simulink model "buck_boost_DCDC_sim"  (R2020a)
settings: Solver=FixedStepAuto  StartTime=0.0  StopTime=sim_duration  FixedStep=time_step  RelTol=1e-3
undefined symbols (not defined in the file): beta, C, E, K_fl, K_smc_0, L, noise_enable, phi, prefiltar_enable, R, R_dot_enable, sigma_noise, step_poremecaj, step_ref, t_poremecaj, t_ref, time_step, w_diff, w_prefiltar, x_2e
settings Model: Creator=HP  LastModifiedBy=HP

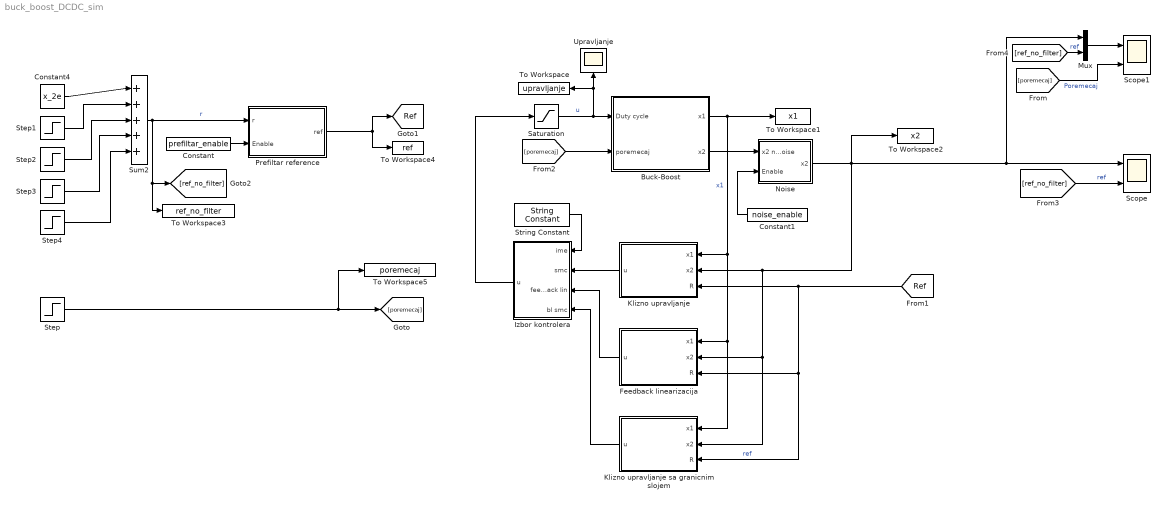
== system buck_boost_DCDC_sim ==
  Buck-Boost : Subsystem
  Constant : Constant  Value=prefiltar_enable
  Constant1 : Constant  Value=noise_enable
  Constant4 : Constant  Value=x_2e
  Feedback linearizacija : Subsystem
  Izbor kontrolera : Subsystem
  Klizno upravljanje : Subsystem
  Klizno upravljanje sa granicnim slojem : Subsystem
  Mux : Mux  Inputs=2
  Noise : Subsystem
  Prefiltar reference : Subsystem
  Saturation : Saturate  UpperLimit=1  LowerLimit=0
  Scope : Scope  NumInputPorts=2
  Scope1 : Scope  NumInputPorts=2
  Step : Step  Time=t_poremecaj(1)  After=step_poremecaj(1)  SampleTime=0
  Step1 : Step  Time=t_ref(1)  After=step_ref(1)  SampleTime=0
  Step2 : Step  Time=t_ref(2)  After=step_ref(2)  SampleTime=0
  Step3 : Step  Time=t_ref(3)  After=step_ref(3)  SampleTime=0
  Step4 : Step  Time=t_ref(4)  After=step_ref(4)  SampleTime=0
  String Constant : StringConstant  String=ime_kontrolera
  Sum2 : Sum  Inputs=|+++++
  To Workspace : ToWorkspace  VariableName=upravljanje  SaveFormat=Timeseries  SampleTime=-1
  To Workspace1 : ToWorkspace  VariableName=x1  SaveFormat=Timeseries  SampleTime=-1
  To Workspace2 : ToWorkspace  VariableName=x2  SaveFormat=Timeseries  SampleTime=-1
  To Workspace3 : ToWorkspace  VariableName=ref_no_filter  SaveFormat=Timeseries  SampleTime=-1
  To Workspace4 : ToWorkspace  VariableName=ref  SaveFormat=Timeseries  SampleTime=-1
  To Workspace5 : ToWorkspace  VariableName=poremecaj  SaveFormat=Timeseries  SampleTime=-1
  Upravljanje : Scope
  tag scope: Ref=global
  wires:
  [ref_no_filter] -> Scope/2  "ref"
  Step1/1 -> Sum2/2
  Constant4/1 -> Sum2/1
  Saturation/1 -> Buck-Boost/1(Duty cycle), To Workspace/1, Upravljanje/1  "u"
  Step2/1 -> Sum2/3
  Buck-Boost/1(x1) -> Klizno upravljanje sa granicnim slojem/1(x1), Feedback linearizacija/1(x1), Klizno upravljanje/1(x1), To Workspace1/1  "x1"
  [Ref] -> Klizno upravljanje sa granicnim slojem/3(R), Feedback linearizacija/3(R), Klizno upravljanje/3(R)  "ref"
  Step/1 -> To Workspace5/1, [poremecaj]
  [poremecaj] -> Buck-Boost/2(poremecaj)
  Sum2/1 -> Prefiltar reference/1(r), [ref_no_filter], To Workspace3/1  "r"
  String Constant/1 -> Izbor kontrolera/1(ime)
  Izbor kontrolera/1(u) -> Saturation/1
  Klizno upravljanje/1(u) -> Izbor kontrolera/2(smc)
  Feedback linearizacija/1(u) -> Izbor kontrolera/3(feedback lin)
  Klizno upravljanje sa granicnim slojem/1(u) -> Izbor kontrolera/4(bl smc)
  Step3/1 -> Sum2/4
  Step4/1 -> Sum2/5
  Mux/1 -> Scope1/1
  [ref_no_filter] -> Mux/2  "ref"
  [poremecaj] -> Scope1/2  "Poremecaj"
  Noise/1(x2) -> Mux/1, Scope/1, To Workspace2/1, Klizno upravljanje sa granicnim slojem/2(x2), Feedback linearizacija/2(x2), Klizno upravljanje/2(x2)
  Buck-Boost/2(x2) -> Noise/1(x2 no noise)
  Constant1/1 -> Noise/2(Enable)
  Prefiltar reference/1(ref) -> [Ref], To Workspace4/1
  Constant/1 -> Prefiltar reference/2(Enable)

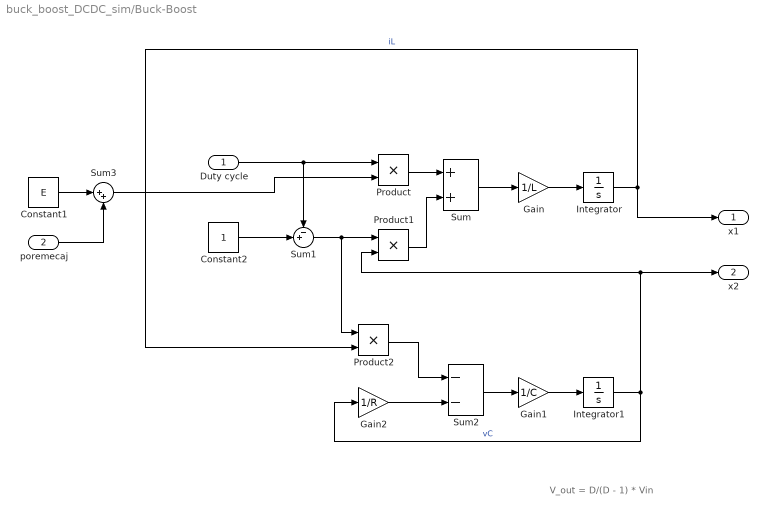
== system buck_boost_DCDC_sim/Buck-Boost ==
  note: V_out = D/(D - 1) * Vin
  Duty cycle : Inport
  poremecaj : Inport  Port=2
  Constant1 : Constant  Value=E
  Constant2 : Constant
  Gain : Gain  Gain=1/L
  Gain1 : Gain  Gain=1/C
  Gain2 : Gain  Gain=1/R
  Integrator : Integrator  InitialCondition=1e-3
  Integrator1 : Integrator  InitialCondition=-1e-3
  Product : Product
  Product1 : Product
  Product2 : Product
  Sum : Sum
  Sum1 : Sum  Inputs=-+|
  Sum2 : Sum  Inputs=--
  Sum3 : Sum  Inputs=|++
  x1 : Outport
  x2 : Outport  Port=2
  wires:
  Product/1 -> Sum/1
  Product1/1 -> Sum/2
  Sum2/1 -> Gain1/1
  Integrator1/1 -> Gain2/1, x2/1, Product1/2  "vC"
  Gain1/1 -> Integrator1/1
  Constant2/1 -> Sum1/2
  Integrator/1 -> x1/1, Product2/2  "iL"
  Sum/1 -> Gain/1
  Gain2/1 -> Sum2/2
  Sum1/1 -> Product2/1, Product1/1
  Duty cycle/1 -> Sum1/1, Product/1
  Product2/1 -> Sum2/1
  Gain/1 -> Integrator/1
  Constant1/1 -> Sum3/1
  Sum3/1 -> Product/2
  poremecaj/1 -> Sum3/2

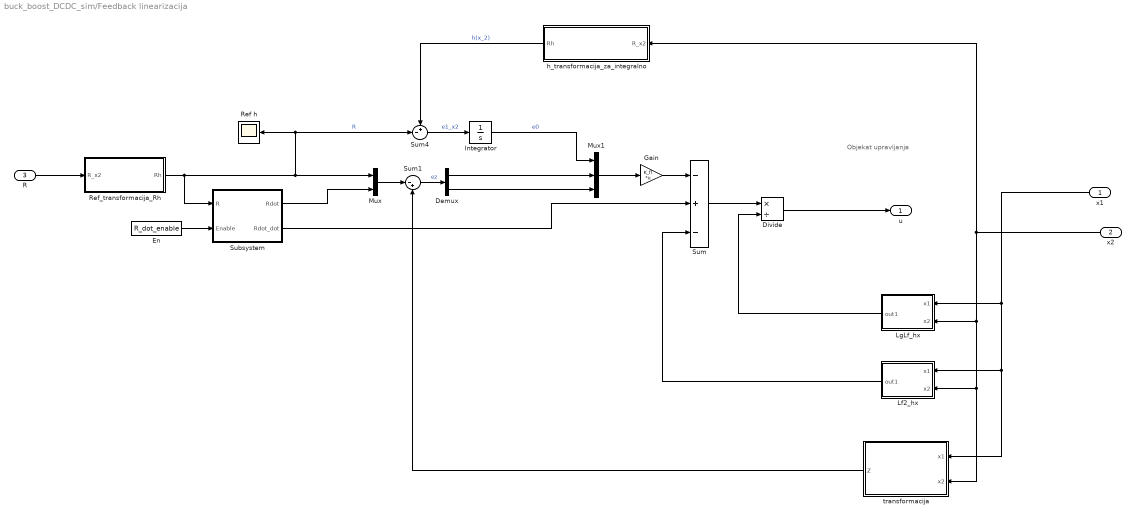
== system buck_boost_DCDC_sim/Feedback linearizacija ==
  note: Objekat upravljanja
  x1 : Inport
  x2 : Inport  Port=2
  R : Inport  Port=3
  Demux : Demux  Outputs=2
  Divide : Product  Inputs=*/
  En : Constant  Value=R_dot_enable
  Gain : Gain  Gain=K_fl  Multiplication=Matrix(K*u)
  Integrator : Integrator
  Lf2_hx : MATLAB Function  TreatAsAtomicUnit=on
  LgLf_hx : MATLAB Function  TreatAsAtomicUnit=on
  Mux : Mux  Inputs=2
  Mux1 : Mux  Inputs=3
  Ref h : Scope
  Ref_transformacija_Rh : MATLAB Function  TreatAsAtomicUnit=on
  Subsystem : Subsystem
  Sum : Sum  Inputs=-+-
  Sum1 : Sum  Inputs=|-+
  Sum4 : Sum  Inputs=+-|
  h_transformacija_za_integralno : MATLAB Function  TreatAsAtomicUnit=on
  transformacija : MATLAB Function  TreatAsAtomicUnit=on
  u : Outport
  wires:
  Subsystem/1(Rdot) -> Mux/2
  Divide/1 -> u/1
  Ref_transformacija_Rh/1(Rh) -> Sum4/2, Ref h/1, Mux/1, Subsystem/1(R)  "R"
  x1/1 -> LgLf_hx/1(x1), Lf2_hx/1(x1), transformacija/1(x1)
  Mux/1 -> Sum1/1
  LgLf_hx/1(out1) -> Divide/2
  x2/1 -> h_transformacija_za_integralno/1(R_x2), LgLf_hx/2(x2), Lf2_hx/2(x2), transformacija/2(x2)
  Demux/1 -> Mux1/2
  Sum1/1 -> Demux/1  "ez"
  Gain/1 -> Sum/1
  Subsystem/2(Rdot_dot) -> Sum/2
  Lf2_hx/1(out1) -> Sum/3
  En/1 -> Subsystem/2(Enable)
  transformacija/1(Z) -> Sum1/2
  R/1 -> Ref_transformacija_Rh/1(R_x2)
  Sum/1 -> Divide/1
  Mux1/1 -> Gain/1
  Integrator/1 -> Mux1/1  "e0"
  Sum4/1 -> Integrator/1  "e1_x2"
  Demux/2 -> Mux1/3
  h_transformacija_za_integralno/1(Rh) -> Sum4/1  "h(x_2)"

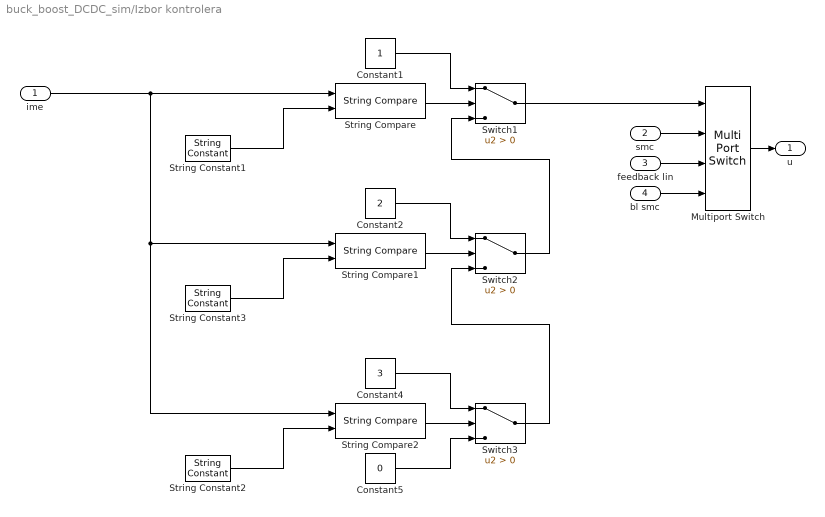
== system buck_boost_DCDC_sim/Izbor kontrolera ==
  ime : Inport
  smc : Inport  Port=2
  feedback lin : Inport  Port=3
  bl smc : Inport  Port=4
  Constant1 : Constant
  Constant2 : Constant  Value=2
  Constant4 : Constant  Value=3
  Constant5 : Constant  Value=0
  Multiport Switch : MultiPortSwitch
  String Compare : StringCompare
  String Compare1 : StringCompare
  String Compare2 : StringCompare
  String Constant1 : StringConstant  String="\"smc\""
  String Constant2 : StringConstant  String="\"bl smc\""
  String Constant3 : StringConstant  String="\"fbl\""
  Switch1 : Switch  Criteria=u2 > Threshold
  Switch2 : Switch  Criteria=u2 > Threshold
  Switch3 : Switch  Criteria=u2 > Threshold
  u : Outport
  wires:
  String Compare1/1 -> Switch2/2
  Switch1/1 -> Multiport Switch/1
  String Constant1/1 -> String Compare/2
  String Constant3/1 -> String Compare1/2
  Constant1/1 -> Switch1/1
  Constant2/1 -> Switch2/1
  Switch2/1 -> Switch1/3
  String Compare/1 -> Switch1/2
  feedback lin/1 -> Multiport Switch/3
  Multiport Switch/1 -> u/1
  smc/1 -> Multiport Switch/2
  bl smc/1 -> Multiport Switch/4
  Constant5/1 -> Switch3/3
  ime/1 -> String Compare/1, String Compare2/1, String Compare1/1
  String Compare2/1 -> Switch3/2
  String Constant2/1 -> String Compare2/2
  Constant4/1 -> Switch3/1
  Switch3/1 -> Switch2/3

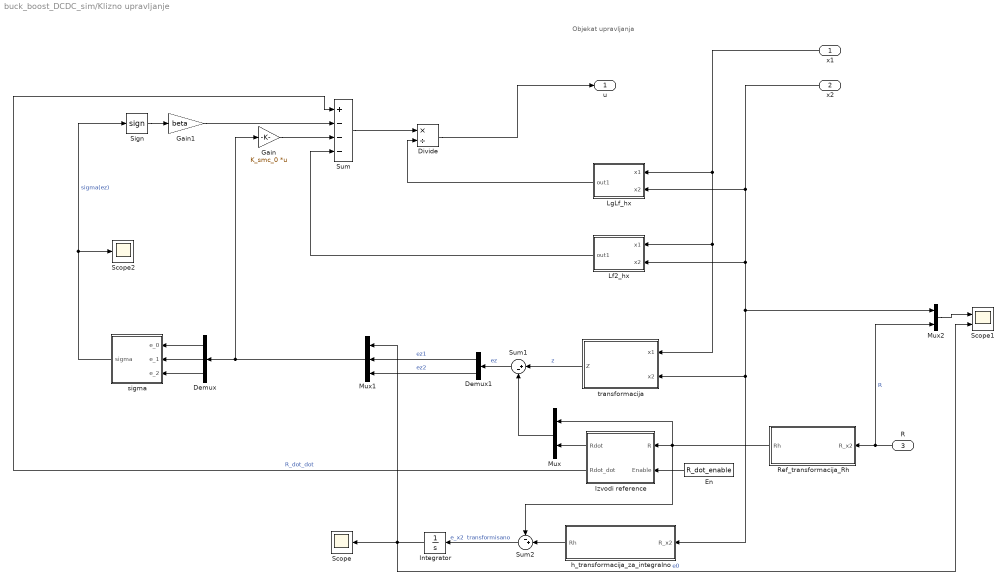
== system buck_boost_DCDC_sim/Klizno upravljanje ==
  note: Objekat upravljanja
  x1 : Inport
  x2 : Inport  Port=2
  R : Inport  Port=3
  Demux : Demux  Outputs=3
  Demux1 : Demux  Outputs=2
  Divide : Product  Inputs=*/
  En : Constant  Value=R_dot_enable
  Gain : Gain  Gain=K_smc_0  Multiplication=Matrix(K*u)
  Gain1 : Gain  Gain=beta
  Integrator : Integrator
  Izvodi reference : Subsystem
  Lf2_hx : MATLAB Function  TreatAsAtomicUnit=on
  LgLf_hx : MATLAB Function  TreatAsAtomicUnit=on
  Mux : Mux  Inputs=2
  Mux1 : Mux  Inputs=3
  Mux2 : Mux  Inputs=2
  Ref_transformacija_Rh : MATLAB Function  TreatAsAtomicUnit=on
  Scope : Scope
  Scope1 : Scope  NumInputPorts=2
  Scope2 : Scope
  Sign : Signum
  Sum : Sum  Inputs=+---
  Sum1 : Sum  Inputs=|+-
  Sum2 : Sum  Inputs=-+|
  h_transformacija_za_integralno : MATLAB Function  TreatAsAtomicUnit=on
  sigma : MATLAB Function  TreatAsAtomicUnit=on
  transformacija : MATLAB Function  TreatAsAtomicUnit=on
  u : Outport
  wires:
  x1/1 -> LgLf_hx/1(x1), transformacija/1(x1), Lf2_hx/1(x1)
  x2/1 -> Mux2/1, h_transformacija_za_integralno/1(R_x2), transformacija/2(x2), Lf2_hx/2(x2), LgLf_hx/2(x2)
  Divide/1 -> u/1
  LgLf_hx/1(out1) -> Divide/2
  Sum/1 -> Divide/1
  Lf2_hx/1(out1) -> Sum/4
  Gain/1 -> Sum/3
  transformacija/1(Z) -> Sum1/1  "z"
  sigma/1(sigma) -> Sign/1, Scope2/1  "sigma(ez)"
  Sign/1 -> Gain1/1
  Gain1/1 -> Sum/2
  En/1 -> Izvodi reference/2(Enable)
  R/1 -> Mux2/2, Ref_transformacija_Rh/1(R_x2)  "R"
  Izvodi reference/1(Rdot) -> Mux/2
  Mux/1 -> Sum1/2
  Izvodi reference/2(Rdot_dot) -> Sum/1  "R_dot_dot"
  Ref_transformacija_Rh/1(Rh) -> Sum2/1, Mux/1, Izvodi reference/1(R)
  Mux1/1 -> Gain/1, Demux/1
  Sum1/1 -> Demux1/1  "ez"
  Demux1/1 -> Mux1/2  "ez1"
  Demux1/2 -> Mux1/3  "ez2"
  h_transformacija_za_integralno/1(Rh) -> Sum2/2
  Sum2/1 -> Integrator/1  "e_x2  transformisano"
  Demux/1 -> sigma/1(e_0)
  Demux/2 -> sigma/2(e_1)
  Demux/3 -> sigma/3(e_2)
  Integrator/1 -> Scope1/2, Scope/1, Mux1/1  "e0"
  Mux2/1 -> Scope1/1

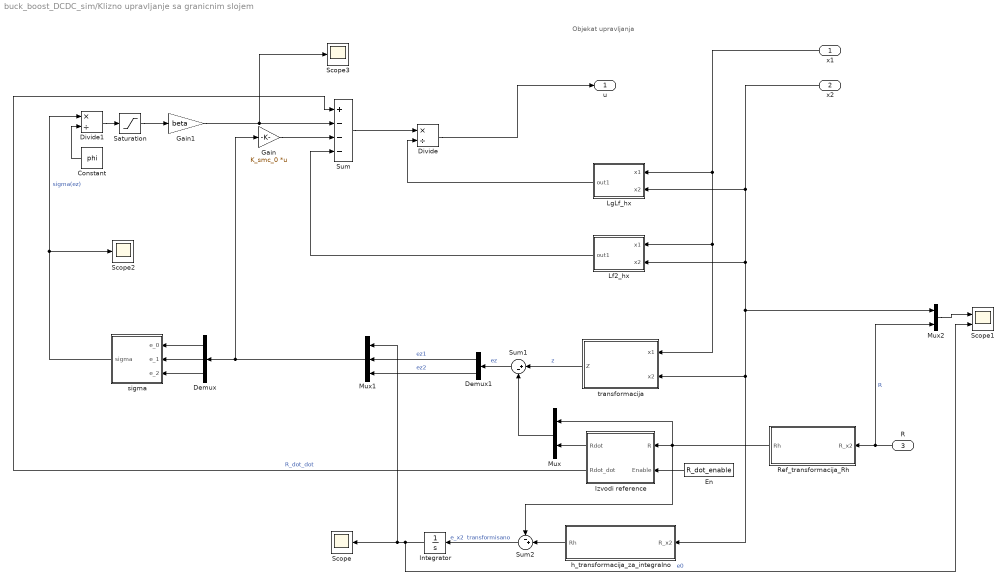
== system buck_boost_DCDC_sim/Klizno upravljanje sa granicnim slojem ==
  note: Objekat upravljanja
  x1 : Inport
  x2 : Inport  Port=2
  R : Inport  Port=3
  Constant : Constant  Value=phi
  Demux : Demux  Outputs=3
  Demux1 : Demux  Outputs=2
  Divide : Product  Inputs=*/
  Divide1 : Product  Inputs=*/
  En : Constant  Value=R_dot_enable
  Gain : Gain  Gain=K_smc_0  Multiplication=Matrix(K*u)
  Gain1 : Gain  Gain=beta
  Integrator : Integrator
  Izvodi reference : Subsystem
  Lf2_hx : MATLAB Function  TreatAsAtomicUnit=on
  LgLf_hx : MATLAB Function  TreatAsAtomicUnit=on
  Mux : Mux  Inputs=2
  Mux1 : Mux  Inputs=3
  Mux2 : Mux  Inputs=2
  Ref_transformacija_Rh : MATLAB Function  TreatAsAtomicUnit=on
  Saturation : Saturate  UpperLimit=1  LowerLimit=-1
  Scope : Scope
  Scope1 : Scope  NumInputPorts=2
  Scope2 : Scope
  Scope3 : Scope
  Sum : Sum  Inputs=+---
  Sum1 : Sum  Inputs=|+-
  Sum2 : Sum  Inputs=-+|
  h_transformacija_za_integralno : MATLAB Function  TreatAsAtomicUnit=on
  sigma : MATLAB Function  TreatAsAtomicUnit=on
  transformacija : MATLAB Function  TreatAsAtomicUnit=on
  u : Outport
  wires:
  x1/1 -> LgLf_hx/1(x1), transformacija/1(x1), Lf2_hx/1(x1)
  x2/1 -> Mux2/1, h_transformacija_za_integralno/1(R_x2), transformacija/2(x2), Lf2_hx/2(x2), LgLf_hx/2(x2)
  Divide/1 -> u/1
  LgLf_hx/1(out1) -> Divide/2
  Sum/1 -> Divide/1
  Lf2_hx/1(out1) -> Sum/4
  Gain/1 -> Sum/3
  transformacija/1(Z) -> Sum1/1  "z"
  sigma/1(sigma) -> Divide1/1, Scope2/1  "sigma(ez)"
  Saturation/1 -> Gain1/1
  Gain1/1 -> Scope3/1, Sum/2
  En/1 -> Izvodi reference/2(Enable)
  R/1 -> Mux2/2, Ref_transformacija_Rh/1(R_x2)  "R"
  Izvodi reference/1(Rdot) -> Mux/2
  Mux/1 -> Sum1/2
  Izvodi reference/2(Rdot_dot) -> Sum/1  "R_dot_dot"
  Ref_transformacija_Rh/1(Rh) -> Sum2/1, Mux/1, Izvodi reference/1(R)
  Mux1/1 -> Gain/1, Demux/1
  Sum1/1 -> Demux1/1  "ez"
  Demux1/1 -> Mux1/2  "ez1"
  Demux1/2 -> Mux1/3  "ez2"
  h_transformacija_za_integralno/1(Rh) -> Sum2/2
  Sum2/1 -> Integrator/1  "e_x2  transformisano"
  Demux/1 -> sigma/1(e_0)
  Demux/2 -> sigma/2(e_1)
  Demux/3 -> sigma/3(e_2)
  Integrator/1 -> Scope1/2, Scope/1, Mux1/1  "e0"
  Mux2/1 -> Scope1/1
  Divide1/1 -> Saturation/1
  Constant/1 -> Divide1/2

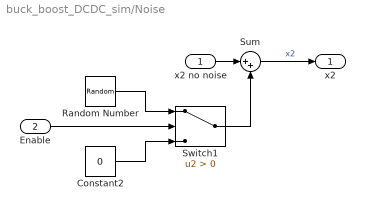
== system buck_boost_DCDC_sim/Noise ==
  x2 no noise : Inport
  Enable : Inport  Port=2
  Constant2 : Constant  Value=0
  Random Number : RandomNumber  Variance=sigma_noise^2  SampleTime=time_step
  Sum : Sum  Inputs=|++
  Switch1 : Switch  Criteria=u2 > Threshold
  x2 : Outport
  wires:
  Random Number/1 -> Switch1/1
  Sum/1 -> x2/1  "x2"
  Switch1/1 -> Sum/2
  Enable/1 -> Switch1/2
  Constant2/1 -> Switch1/3
  x2 no noise/1 -> Sum/1

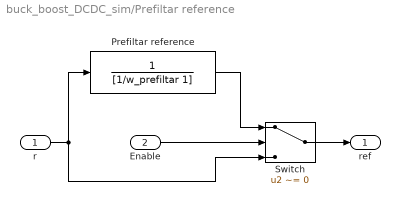
== system buck_boost_DCDC_sim/Prefiltar reference ==
  r : Inport
  Enable : Inport  Port=2
  Prefiltar reference : TransferFcn  Denominator=[1/w_prefiltar 1]
  Switch : Switch  Criteria=u2 ~= 0
  ref : Outport
  wires:
  r/1 -> Switch/3, Prefiltar reference/1
  Enable/1 -> Switch/2
  Switch/1 -> ref/1
  Prefiltar reference/1 -> Switch/1

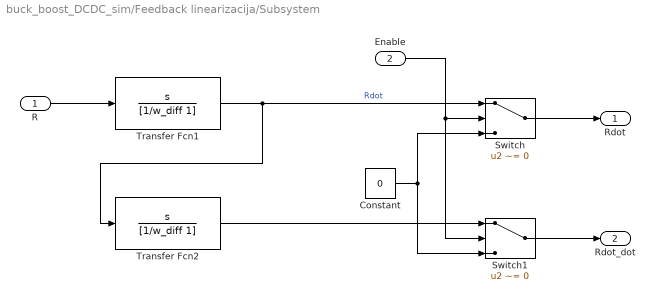
== system buck_boost_DCDC_sim/Feedback linearizacija/Subsystem ==
  R : Inport
  Enable : Inport  Port=2
  Constant : Constant  Value=0
  Switch : Switch  Criteria=u2 ~= 0
  Switch1 : Switch  Criteria=u2 ~= 0
  Transfer Fcn1 : TransferFcn  Numerator=[1 0]  Denominator=[1/w_diff 1]
  Transfer Fcn2 : TransferFcn  Numerator=[1 0]  Denominator=[1/w_diff 1]
  Rdot : Outport
  Rdot_dot : Outport  Port=2
  wires:
  Transfer Fcn1/1 -> Switch/1, Transfer Fcn2/1  "Rdot"
  R/1 -> Transfer Fcn1/1
  Transfer Fcn2/1 -> Switch1/1
  Enable/1 -> Switch1/2, Switch/2
  Constant/1 -> Switch1/3, Switch/3
  Switch/1 -> Rdot/1
  Switch1/1 -> Rdot_dot/1

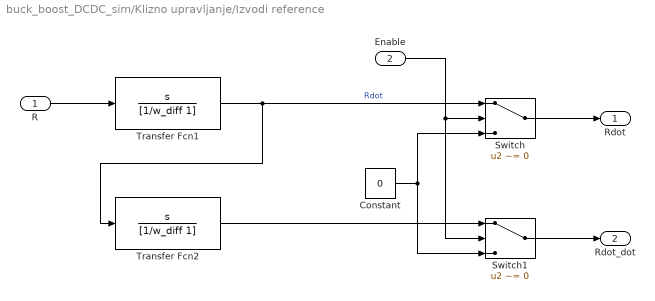
== system buck_boost_DCDC_sim/Klizno upravljanje/Izvodi reference ==
  R : Inport
  Enable : Inport  Port=2
  Constant : Constant  Value=0
  Switch : Switch  Criteria=u2 ~= 0
  Switch1 : Switch  Criteria=u2 ~= 0
  Transfer Fcn1 : TransferFcn  Numerator=[1 0]  Denominator=[1/w_diff 1]
  Transfer Fcn2 : TransferFcn  Numerator=[1 0]  Denominator=[1/w_diff 1]
  Rdot : Outport
  Rdot_dot : Outport  Port=2
  wires:
  Transfer Fcn1/1 -> Switch/1, Transfer Fcn2/1  "Rdot"
  R/1 -> Transfer Fcn1/1
  Transfer Fcn2/1 -> Switch1/1
  Enable/1 -> Switch1/2, Switch/2
  Constant/1 -> Switch1/3, Switch/3
  Switch/1 -> Rdot/1
  Switch1/1 -> Rdot_dot/1

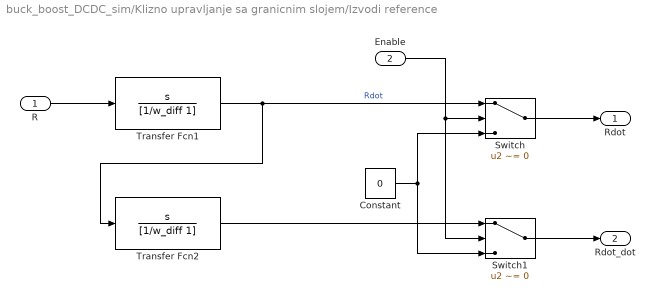
== system buck_boost_DCDC_sim/Klizno upravljanje sa granicnim slojem/Izvodi reference ==
  R : Inport
  Enable : Inport  Port=2
  Constant : Constant  Value=0
  Switch : Switch  Criteria=u2 ~= 0
  Switch1 : Switch  Criteria=u2 ~= 0
  Transfer Fcn1 : TransferFcn  Numerator=[1 0]  Denominator=[1/w_diff 1]
  Transfer Fcn2 : TransferFcn  Numerator=[1 0]  Denominator=[1/w_diff 1]
  Rdot : Outport
  Rdot_dot : Outport  Port=2
  wires:
  Transfer Fcn1/1 -> Switch/1, Transfer Fcn2/1  "Rdot"
  R/1 -> Transfer Fcn1/1
  Transfer Fcn2/1 -> Switch1/1
  Enable/1 -> Switch1/2, Switch/2
  Constant/1 -> Switch1/3, Switch/3
  Switch/1 -> Rdot/1
  Switch1/1 -> Rdot_dot/1

== matlab function buck_boost_DCDC_sim/Klizno upravljanje sa granicnim slojem/LgLf_hx ==
  data: x1 input; out1 output; x2 input
function out1 = LgLf_hx(x1,x2)
%#codegen

%    This function was generated by the Symbolic Math Toolbox version 8.5.
%    18-Dec-2020 13:49:38

out1 = x1.*9.819967266775777e+2-x2.*1.508485229415462e+3-x1.*x2.*1.636661211129296e+2+1.810182275298554e+4;

== matlab function buck_boost_DCDC_sim/Klizno upravljanje sa granicnim slojem/Ref_transformacija_Rh ==
  data: R_x2 input; Rh output
function Rh = Ref_transformacija_Rh(R_x2)
%#codegen

%    This function was generated by the Symbolic Math Toolbox version 8.5.
%    18-Dec-2020 13:49:39

t2 = R_x2.^2;
Rh = R_x2.*(-1.128e-2)+t2.*4.7e-4+(R_x2.*1.2e+1-t2).^2.*4.086024819197896e-8-5.163584171453171e-1;

== matlab function buck_boost_DCDC_sim/Klizno upravljanje sa granicnim slojem/h_transformacija_za_integralno ==
  data: R_x2 input; Rh output
function Rh = h_transformacija_za_integralno(R_x2)
%#codegen

%    This function was generated by the Symbolic Math Toolbox version 8.5.
%    18-Dec-2020 13:49:39

t2 = R_x2.^2;
Rh = R_x2.*(-1.128e-2)+t2.*4.7e-4+(R_x2.*1.2e+1-t2).^2.*4.086024819197896e-8-5.163584171453171e-1;

== matlab function buck_boost_DCDC_sim/Klizno upravljanje sa granicnim slojem/sigma ==
  data: sigma output; e_0 input; e_1 input; e_2 input
function sigma = sigma(e_0,e_1,e_2)
%#codegen

%    This function was generated by the Symbolic Math Toolbox version 8.5.
%    18-Dec-2020 13:49:39

sigma = e_0.*9.0e+4+e_1.*6.0e+2+e_2;

== matlab function buck_boost_DCDC_sim/Klizno upravljanje sa granicnim slojem/transformacija ==
  data: Z output; x1 input; x2 input
function Z = transformacija(x1,x2)
%#codegen

%    This function was generated by the Symbolic Math Toolbox version 8.5.
%    18-Dec-2020 13:49:38

Z = [x2.*(-1.128e-2)+x1.^2.*1.591e-2+x2.^2.*4.7e-4-5.163584171453171e-1;(x2.*9.4e-4-1.128e-2).*(x1.*5.2e+1+x2).*(-4.091653027823241e+1)+x1.*x2.*2.0];

== matlab function buck_boost_DCDC_sim/Feedback linearizacija/LgLf_hx ==
  data: x1 input; out1 output; x2 input
function out1 = LgLf_hx(x1,x2)
%#codegen

%    This function was generated by the Symbolic Math Toolbox version 8.5.
%    18-Dec-2020 13:49:34

out1 = x1.*9.819967266775777e+2-x2.*1.508485229415462e+3-x1.*x2.*1.636661211129296e+2+1.810182275298554e+4;

== matlab function buck_boost_DCDC_sim/Feedback linearizacija/transformacija ==
  data: x1 input; Z output; x2 input
function Z = transformacija(x1,x2)
%#codegen

%    This function was generated by the Symbolic Math Toolbox version 8.5.
%    18-Dec-2020 13:49:33

Z = [x2.*(-1.128e-2)+x1.^2.*1.591e-2+x2.^2.*4.7e-4-5.163584171453171e-1;(x2.*9.4e-4-1.128e-2).*(x1.*5.2e+1+x2).*(-4.091653027823241e+1)+x1.*x2.*2.0];

== matlab function buck_boost_DCDC_sim/Feedback linearizacija/Lf2_hx ==
  data: x1 input; out1 output; x2 input
function out1 = Lf2_hx(x1,x2)
%#codegen

%    This function was generated by the Symbolic Math Toolbox version 8.5.
%    18-Dec-2020 13:49:34

out1 = x2.*1.508485229415462e+3+(x2./1.3e+1-6.0./1.3e+1).*(x1.*5.2e+1+x2).*4.091653027823241e+1;

== matlab function buck_boost_DCDC_sim/Feedback linearizacija/Ref_transformacija_Rh ==
  data: R_x2 input; Rh output
function Rh = Ref_transformacija_Rh(R_x2)
%#codegen

%    This function was generated by the Symbolic Math Toolbox version 8.5.
%    18-Dec-2020 13:49:34

t2 = R_x2.^2;
Rh = R_x2.*(-1.128e-2)+t2.*4.7e-4+(R_x2.*1.2e+1-t2).^2.*4.086024819197896e-8-5.163584171453171e-1;

== matlab function buck_boost_DCDC_sim/Feedback linearizacija/h_transformacija_za_integralno ==
  data: R_x2 input; Rh output
function Rh = h_transformacija_za_integralno(R_x2)
%#codegen

%    This function was generated by the Symbolic Math Toolbox version 8.5.
%    18-Dec-2020 13:49:34

t2 = R_x2.^2;
Rh = R_x2.*(-1.128e-2)+t2.*4.7e-4+(R_x2.*1.2e+1-t2).^2.*4.086024819197896e-8-5.163584171453171e-1;

== matlab function buck_boost_DCDC_sim/Klizno upravljanje/transformacija ==
  data: Z output; x1 input; x2 input
function Z = transformacija(x1,x2)
%#codegen

%    This function was generated by the Symbolic Math Toolbox version 8.5.
%    18-Dec-2020 13:49:36

Z = [x2.*(-1.128e-2)+x1.^2.*1.591e-2+x2.^2.*4.7e-4-5.163584171453171e-1;(x2.*9.4e-4-1.128e-2).*(x1.*5.2e+1+x2).*(-4.091653027823241e+1)+x1.*x2.*2.0];

== matlab function buck_boost_DCDC_sim/Klizno upravljanje/LgLf_hx ==
  data: x1 input; out1 output; x2 input
function out1 = LgLf_hx(x1,x2)
%#codegen

%    This function was generated by the Symbolic Math Toolbox version 8.5.
%    18-Dec-2020 13:49:36

out1 = x1.*9.819967266775777e+2-x2.*1.508485229415462e+3-x1.*x2.*1.636661211129296e+2+1.810182275298554e+4;

== matlab function buck_boost_DCDC_sim/Klizno upravljanje/Lf2_hx ==
  data: x1 input; out1 output; x2 input
function out1 = Lf2_hx(x1,x2)
%#codegen

%    This function was generated by the Symbolic Math Toolbox version 8.5.
%    18-Dec-2020 13:49:36

out1 = x2.*1.508485229415462e+3+(x2./1.3e+1-6.0./1.3e+1).*(x1.*5.2e+1+x2).*4.091653027823241e+1;

== matlab function buck_boost_DCDC_sim/Klizno upravljanje/sigma ==
  data: sigma output; e_0 input; e_1 input; e_2 input
function sigma = sigma(e_0,e_1,e_2)
%#codegen

%    This function was generated by the Symbolic Math Toolbox version 8.5.
%    18-Dec-2020 13:49:37

sigma = e_0.*9.0e+4+e_1.*6.0e+2+e_2;

== matlab function buck_boost_DCDC_sim/Klizno upravljanje/Ref_transformacija_Rh ==
  data: R_x2 input; Rh output
function Rh = Ref_transformacija_Rh(R_x2)
%#codegen

%    This function was generated by the Symbolic Math Toolbox version 8.5.
%    18-Dec-2020 13:49:37

t2 = R_x2.^2;
Rh = R_x2.*(-1.128e-2)+t2.*4.7e-4+(R_x2.*1.2e+1-t2).^2.*4.086024819197896e-8-5.163584171453171e-1;

== matlab function buck_boost_DCDC_sim/Klizno upravljanje/h_transformacija_za_integralno ==
  data: R_x2 input; Rh output
function Rh = h_transformacija_za_integralno(R_x2)
%#codegen

%    This function was generated by the Symbolic Math Toolbox version 8.5.
%    18-Dec-2020 13:49:37

t2 = R_x2.^2;
Rh = R_x2.*(-1.128e-2)+t2.*4.7e-4+(R_x2.*1.2e+1-t2).^2.*4.086024819197896e-8-5.163584171453171e-1;

== matlab function buck_boost_DCDC_sim/Klizno upravljanje sa granicnim slojem/Lf2_hx ==
  data: x1 input; out1 output; x2 input
function out1 = Lf2_hx(x1,x2)
%#codegen

%    This function was generated by the Symbolic Math Toolbox version 8.5.
%    18-Dec-2020 13:49:39

out1 = x2.*1.508485229415462e+3+(x2./1.3e+1-6.0./1.3e+1).*(x1.*5.2e+1+x2).*4.091653027823241e+1;
